simulink model "CAL_TITA_L"  (R2024b)
settings: Solver=VariableStepAuto  StartTime=0.0  StopTime=10.0  RelTol=1e-3
undefined symbols (not defined in the file): Yt0
settings Model: Creator=Ignacio  LastModifiedBy=ribei
settings RTWCC: GPUComputeCapability=3.5

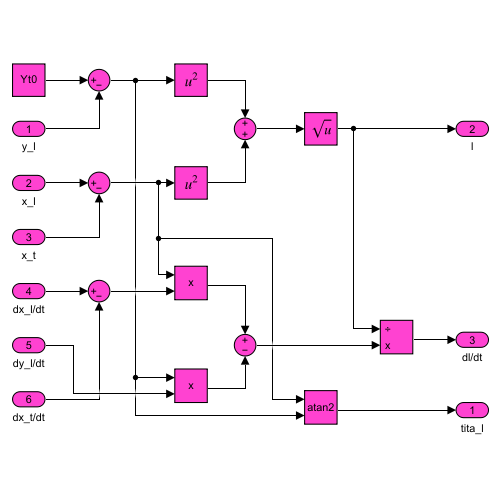
[thumbnail: Simulink's stored preview of the top-level diagram]
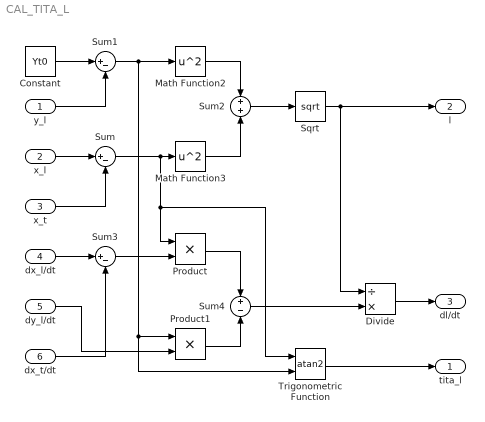
== system CAL_TITA_L ==
  y_l : Inport
  x_l : Inport  Port=2
  x_t : Inport  Port=3
  dx_l/dt : Inport  Port=4
  dy_l/dt : Inport  Port=5
  dx_t/dt : Inport  Port=6
  Constant : Constant  Value=Yt0
  Divide : Product  Inputs=/*
  Math Function2 : Math  Operator=square
  Math Function3 : Math  Operator=square
  Product : Product
  Product1 : Product
  Sqrt : Sqrt
  Sum : Sum  Inputs=|+-
  Sum1 : Sum  Inputs=|+-
  Sum2 : Sum  Inputs=+|+
  Sum3 : Sum  Inputs=|+-
  Sum4 : Sum  Inputs=+|-
  Trigonometric Function : Trigonometry  Operator=atan2
  tita_l : Outport
  l : Outport  Port=2
  dl/dt : Outport  Port=3
  wires:
  x_l/1 -> Sum/1
  x_t/1 -> Sum/2
  Sum/1 -> Product/1, Trigonometric Function/1, Math Function3/1
  Constant/1 -> Sum1/1
  y_l/1 -> Sum1/2
  Sum1/1 -> Product1/1, Trigonometric Function/2, Math Function2/1
  Math Function2/1 -> Sum2/1
  Math Function3/1 -> Sum2/2
  Sum2/1 -> Sqrt/1
  Sqrt/1 -> l/1, Divide/1
  Divide/1 -> dl/dt/1
  dx_l/dt/1 -> Sum3/1
  dx_t/dt/1 -> Sum3/2
  Sum3/1 -> Product/2
  dy_l/dt/1 -> Product1/2
  Product/1 -> Sum4/1
  Product1/1 -> Sum4/2
  Sum4/1 -> Divide/2
  Trigonometric Function/1 -> tita_l/1
